simulink model "W3P2"  (R2020b)
settings: Solver=VariableStepAuto  StartTime=0.0  StopTime=10.0  RelTol=1e-3
settings Model: EnablePacing=on  PacingRate=0.700000  Creator=ASUS  LastModifiedBy=ASUS

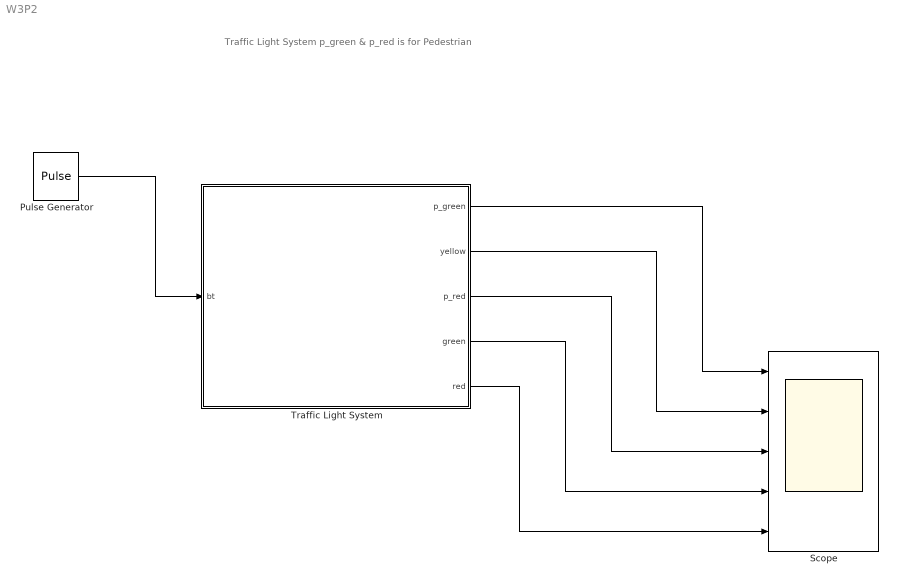
== system W3P2 ==
  note: Traffic Light System
      | p_green & p_red is for Pedestrian
  Pulse Generator : DiscretePulseGenerator  PulseType=Time based  Period=10  PulseWidth=5
  Scope : Scope  NumInputPorts=5
  Traffic Light System : Stateflow chart  TreatAsAtomicUnit=on
  wires:
  Traffic Light System/1(p_green) -> Scope/1
  Traffic Light System/2(yellow) -> Scope/2
  Traffic Light System/3(p_red) -> Scope/3
  Traffic Light System/4(green) -> Scope/4
  Traffic Light System/5(red) -> Scope/5
  Pulse Generator/1 -> Traffic Light System/1(bt)

== stateflow chart W3P2/Traffic Light System ==
  state Start
    entry: p_red=1;
    entry: green=1;
    exit: green=0;
  state up1
    entry: yellow=1;
    exit: yellow=0;
  state up2
    entry: red=1;
    exit: p_red=0;
  state up3
    entry: p_green=1;
  note: p_green & p_red is for Pedestrian
  state blink
    entry:n=0;
    during: n=n+1;
    state w
      entry: p_green=1;
    state nw
      entry: p_green=0;
    (default) -> w
    w -> nw : [after(0.25,sec)]
    nw -> w : [after(0.25,sec)]
  state exit
    exit: red=0;
    exit: p_green=0;
  state up4
    entry: p_red=1;
    entry: yellow=1;
    exit: p_red=0;
    exit: yellow=0;
  (default) -> Start
  up4 -> Start : [after(2,sec)]
  up3 -> blink : [after(5,sec)]
  Start -> up1 : [bt==1]
  up1 -> up2
  up2 -> up3 : [after(1,sec)]
  exit -> up4
  blink -> exit : [n>=9]
  data: bt input; p_green output; yellow output; p_red output; green output; red output; n local
